simulink model "common"  (R2018a)
settings: Solver=VariableStepAuto  StartTime=0.0  StopTime=30  RelTol=1e-3
settings Model: Creator=User  LastModifiedBy=User

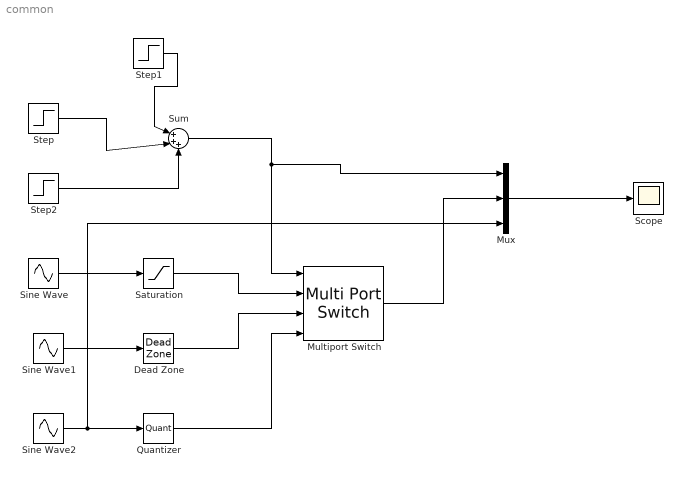
== system common ==
  Dead Zone : DeadZone  SaturateOnIntegerOverflow=on
  Multiport Switch : MultiPortSwitch
  Mux : Mux  Inputs=3
  Quantizer : Quantizer
  Saturation : Saturate
  Scope : Scope
  Sine Wave : Sin  Amplitude=2  SampleTime=0
  Sine Wave1 : Sin  Amplitude=2  SampleTime=0
  Sine Wave2 : Sin  Amplitude=2  SampleTime=0
  Step : Step  Time=7  SampleTime=0
  Step1 : Step  Time=0  SampleTime=0
  Step2 : Step  Time=14  SampleTime=0
  Sum : Sum  Inputs=|+++
  wires:
  Sine Wave/1 -> Saturation/1
  Sine Wave1/1 -> Dead Zone/1
  Dead Zone/1 -> Multiport Switch/3
  Saturation/1 -> Multiport Switch/2
  Sum/1 -> Mux/1, Multiport Switch/1
  Step1/1 -> Sum/1
  Step/1 -> Sum/2
  Step2/1 -> Sum/3
  Quantizer/1 -> Multiport Switch/4
  Multiport Switch/1 -> Mux/2
  Sine Wave2/1 -> Mux/3, Quantizer/1
  Mux/1 -> Scope/1
